simulink library "VIS_LIB"  (Simulink 8.6)
settings: Solver=ode45  StartTime=0.0  StopTime=10.0  RelTol=1e-3
undefined symbols (not defined in the file): AC, SIXOSEM_F_WD_AC_MASTER
libraries: cdsFilt x376, cdsEpicsOut x253, cdsEpicsIn x179, cdsTP x123, VIS_LIB x95, cdsMuxMatrix x91, cdsEpicsStringIn x75, cdsFiltCtrl x72, cdsFunctionCall x70, cdsRms x59, KAGRA_UTIL x25, STATE_BIO_MASTER x5
(part 17 of 38)

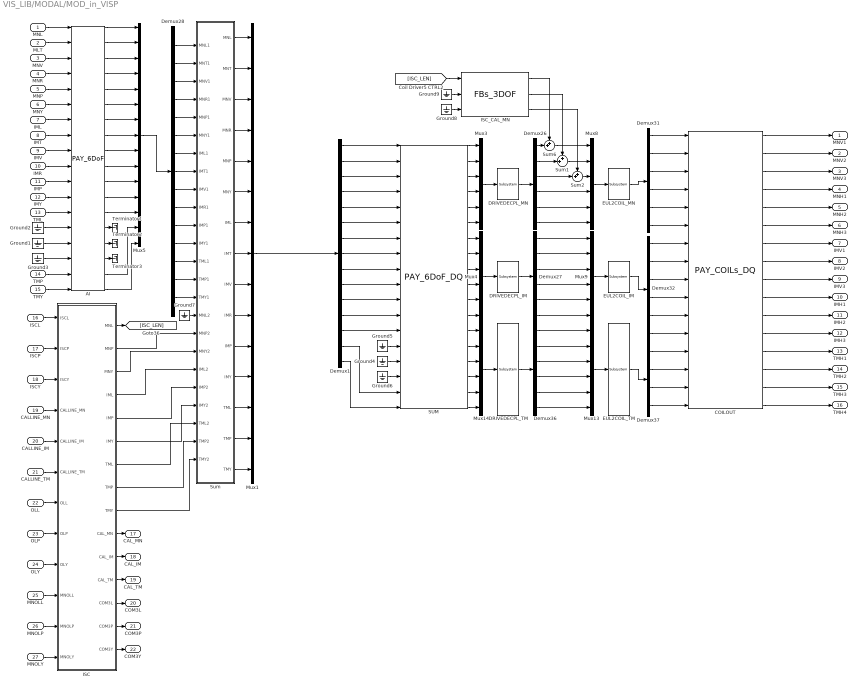
== system VIS_LIB/MODAL/MOD_in_VISP ==
  MNL : Inport
  MLT : Inport  Port=2
  MNV : Inport  Port=3
  MNR : Inport  Port=4
  MNP : Inport  Port=5
  MNY : Inport  Port=6
  IML : Inport  Port=7
  IMT : Inport  Port=8
  IMV : Inport  Port=9
  IMR : Inport  Port=10
  IMP : Inport  Port=11
  IMY : Inport  Port=12
  TML : Inport  Port=13
  TMP : Inport  Port=14
  TMY : Inport  Port=15
  ISCL : Inport  Port=16
  ISCP : Inport  Port=17
  ISCY : Inport  Port=18
  CALLINE_MN : Inport  Port=19
  CALLINE_IM : Inport  Port=20
  CALLINE_TM : Inport  Port=21
  OLL : Inport  Port=22
  OLP : Inport  Port=23
  OLY : Inport  Port=24
  MNOLL : Inport  Port=25
  MNOLP : Inport  Port=26
  MNOLY : Inport  Port=27
  AI : VIS_LIB/UTILs/PAY_6DoF
  COILOUT : VIS_LIB/UTILs/PAY_COILs_DQ
  DRIVEDECPL_IM : cdsMuxMatrix/Subsystem  Tag=cdsMuxMatrix  Description=Any size matrix. Inputs and outputs must be connected using Mux and Demux parts.
      settings: AttributesFormatString=%<Tag>
  DRIVEDECPL_MN : cdsMuxMatrix/Subsystem  Tag=cdsMuxMatrix  Description=Any size matrix. Inputs and outputs must be connected using Mux and Demux parts.
      settings: AttributesFormatString=%<Tag>
  DRIVEDECPL_TM : cdsMuxMatrix/Subsystem  Tag=cdsMuxMatrix  Description=Any size matrix. Inputs and outputs must be connected using Mux and Demux parts.
      settings: AttributesFormatString=%<Tag>
  Demux1 : Demux  Outputs=15
  Demux{26..27,31..32,36} (5 alike) : Demux  Outputs=6
  Demux28 : Demux  Outputs=15
  Demux37 : Demux
  EUL2COIL_IM : cdsMuxMatrix/Subsystem  Tag=cdsMuxMatrix  Description=Any size matrix. Inputs and outputs must be connected using Mux and Demux parts.
      settings: AttributesFormatString=%<Tag>
  EUL2COIL_MN : cdsMuxMatrix/Subsystem  Tag=cdsMuxMatrix  Description=Any size matrix. Inputs and outputs must be connected using Mux and Demux parts.
      settings: AttributesFormatString=%<Tag>
  EUL2COIL_TM : cdsMuxMatrix/Subsystem  Tag=cdsMuxMatrix  Description=Any size matrix. Inputs and outputs must be connected using Mux and Demux parts.
      settings: AttributesFormatString=%<Tag>
  Ground{1..9} (9 alike) : Ground
  ISC : Subsystem
  ISC_CAL_MN : VIS_LIB/UTILs/FBs_3DOF
  Mux1 : Mux  Inputs=15
  Mux{3..4,8..9,13..14} (6 alike) : Mux  Inputs=6
  Mux5 : Mux  Inputs=15
  SUM : VIS_LIB/UTILs/PAY_6DoF_DQ
  Sum : Subsystem
  Sum1 : Sum  Inputs=++|
  Sum2 : Sum  Inputs=++|
  Sum6 : Sum  Inputs=++|
  Terminator1 : Terminator
  Terminator2 : Terminator
  Terminator3 : Terminator
  MNV1 : Outport
  MNV2 : Outport  Port=2
  MNV3 : Outport  Port=3
  MNH1 : Outport  Port=4
  MNH2 : Outport  Port=5
  MNH3 : Outport  Port=6
  IMV1 : Outport  Port=7
  IMV2 : Outport  Port=8
  IMV3 : Outport  Port=9
  IMH1 : Outport  Port=10
  IMH2 : Outport  Port=11
  IMH3 : Outport  Port=12
  TMH1 : Outport  Port=13
  TMH2 : Outport  Port=14
  TMH3 : Outport  Port=15
  TMH4 : Outport  Port=16
  CAL_MN : Outport  Port=17
  CAL_IM : Outport  Port=18
  CAL_TM : Outport  Port=19
  COM3L : Outport  Port=20
  COM3P : Outport  Port=21
  COM3Y : Outport  Port=22
  wires:
  ISC/12(CAL_TM) -> CAL_TM/1
  ISC/11(CAL_IM) -> CAL_IM/1
  ISC/10(CAL_MN) -> CAL_MN/1
  Mux1/1 -> Demux1/1
  Demux1/15 -> SUM/18
  Demux1/14 -> SUM/17
  Demux1/13 -> SUM/13
  Demux1/12 -> SUM/12
  Demux1/10 -> SUM/10
  Demux1/9 -> SUM/9
  Demux1/8 -> SUM/8
  Demux1/7 -> SUM/7
  Demux1/6 -> SUM/6
  Demux1/5 -> SUM/5
  Demux1/4 -> SUM/4
  Demux1/3 -> SUM/3
  Demux1/2 -> SUM/2
  Demux1/1 -> SUM/1
  Ground6/1 -> SUM/16
  Ground4/1 -> SUM/15
  Ground5/1 -> SUM/14
  Demux1/11 -> SUM/11
  Sum/15(TMY) -> Mux1/15
  Sum/14(TMP) -> Mux1/14
  Sum/13(TML) -> Mux1/13
  Sum/12(IMY) -> Mux1/12
  Sum/11(IMP) -> Mux1/11
  Sum/10(IMR) -> Mux1/10
  Sum/9(IMV) -> Mux1/9
  Sum/8(IMT) -> Mux1/8
  Sum/7(IML) -> Mux1/7
  Sum/6(MNY) -> Mux1/6
  Sum/5(MNP) -> Mux1/5
  Sum/4(MNR) -> Mux1/4
  Sum/3(MNV) -> Mux1/3
  Sum/2(MNT) -> Mux1/2
  Sum/1(MNL) -> Mux1/1
  ISCY/1 -> ISC/3(ISCY)
  ISCP/1 -> ISC/2(ISCP)
  CALLINE_MN/1 -> ISC/4(CALLINE_MN)
  CALLINE_IM/1 -> ISC/5(CALLINE_IM)
  CALLINE_TM/1 -> ISC/6(CALLINE_TM)
  ISCL/1 -> ISC/1(ISCL)
  ISC/9(TMY) -> Sum/24(TMY2)
  ISC/8(TMP) -> Sum/23(TMP2)
  ISC/7(TML) -> Sum/22(TML2)
  ISC/6(IMY) -> Sum/21(IMY2)
  ISC/5(IMP) -> Sum/20(IMP2)
  ISC/4(IML) -> Sum/19(IML2)
  Mux5/1 -> Demux28/1
  Demux28/15 -> Sum/15(TMY1)
  Demux28/14 -> Sum/14(TMP1)
  Demux28/13 -> Sum/13(TML1)
  Demux28/12 -> Sum/12(IMY1)
  Demux28/11 -> Sum/11(IMP1)
  Demux28/10 -> Sum/10(IMR1)
  Demux28/9 -> Sum/9(IMV1)
  Demux28/8 -> Sum/8(IMT1)
  Demux28/7 -> Sum/7(IML1)
  Demux28/6 -> Sum/6(MNY1)
  Demux28/5 -> Sum/5(MNP1)
  Demux28/4 -> Sum/4(MNR1)
  Demux28/3 -> Sum/3(MNV1)
  Demux28/2 -> Sum/2(MNT1)
  Demux28/1 -> Sum/1(MNL1)
  AI/18 -> Mux5/15
  AI/17 -> Mux5/14
  AI/13 -> Mux5/13
  AI/12 -> Mux5/12
  AI/11 -> Mux5/11
  AI/10 -> Mux5/10
  AI/9 -> Mux5/9
  AI/8 -> Mux5/8
  AI/7 -> Mux5/7
  AI/6 -> Mux5/6
  AI/5 -> Mux5/5
  AI/4 -> Mux5/4
  AI/3 -> Mux5/3
  AI/2 -> Mux5/2
  AI/1 -> Mux5/1
  AI/16 -> Terminator3/1
  AI/15 -> Terminator2/1
  AI/14 -> Terminator1/1
  SUM/10 -> Mux4/4
  SUM/9 -> Mux4/3
  SUM/8 -> Mux4/2
  SUM/7 -> Mux4/1
  SUM/6 -> Mux3/6
  SUM/5 -> Mux3/5
  SUM/4 -> Mux3/4
  SUM/3 -> Mux3/3
  SUM/2 -> Mux3/2
  SUM/1 -> Mux3/1
  SUM/18 -> Mux14/6
  SUM/17 -> Mux14/5
  SUM/16 -> Mux14/4
  SUM/15 -> Mux14/3
  SUM/14 -> Mux14/2
  SUM/13 -> Mux14/1
  SUM/12 -> Mux4/6
  SUM/11 -> Mux4/5
  COILOUT/16 -> TMH4/1
  COILOUT/15 -> TMH3/1
  COILOUT/14 -> TMH2/1
  COILOUT/13 -> TMH1/1
  COILOUT/12 -> IMH3/1
  COILOUT/11 -> IMH2/1
  COILOUT/10 -> IMH1/1
  COILOUT/9 -> IMV3/1
  COILOUT/8 -> IMV2/1
  COILOUT/7 -> IMV1/1
  COILOUT/6 -> MNH3/1
  COILOUT/5 -> MNH2/1
  COILOUT/4 -> MNH1/1
  COILOUT/3 -> MNV3/1
  COILOUT/2 -> MNV2/1
  COILOUT/1 -> MNV1/1
  Demux37/4 -> COILOUT/16
  Demux37/3 -> COILOUT/15
  Demux37/2 -> COILOUT/14
  Demux37/1 -> COILOUT/13
  Demux32/6 -> COILOUT/12
  Demux32/5 -> COILOUT/11
  Demux32/4 -> COILOUT/10
  Demux32/3 -> COILOUT/9
  Demux32/2 -> COILOUT/8
  Demux32/1 -> COILOUT/7
  Demux31/6 -> COILOUT/6
  Demux31/5 -> COILOUT/5
  Demux31/4 -> COILOUT/4
  Demux31/3 -> COILOUT/3
  Demux31/2 -> COILOUT/2
  Demux31/1 -> COILOUT/1
  Ground3/1 -> AI/16
  Ground1/1 -> AI/15
  Ground2/1 -> AI/14
  TMY/1 -> AI/18
  TMP/1 -> AI/17
  TML/1 -> AI/13
  IMY/1 -> AI/12
  IMP/1 -> AI/11
  IMR/1 -> AI/10
  IMV/1 -> AI/9
  IMT/1 -> AI/8
  IML/1 -> AI/7
  MNY/1 -> AI/6
  MNP/1 -> AI/5
  MNR/1 -> AI/4
  MNV/1 -> AI/3
  MLT/1 -> AI/2
  MNL/1 -> AI/1
  Mux3/1 -> DRIVEDECPL_MN/1
  DRIVEDECPL_MN/1 -> Demux26/1
  Mux4/1 -> DRIVEDECPL_IM/1
  DRIVEDECPL_IM/1 -> Demux27/1
  Mux8/1 -> EUL2COIL_MN/1
  EUL2COIL_MN/1 -> Demux31/1
  Demux26/4 -> Mux8/4
  Demux26/5 -> Mux8/5
  Demux26/6 -> Mux8/6
  Mux9/1 -> EUL2COIL_IM/1
  EUL2COIL_IM/1 -> Demux32/1
  Demux27/1 -> Mux9/1
  Demux27/2 -> Mux9/2
  Demux27/3 -> Mux9/3
  Demux27/4 -> Mux9/4
  Demux27/5 -> Mux9/5
  Demux27/6 -> Mux9/6
  Mux14/1 -> DRIVEDECPL_TM/1
  DRIVEDECPL_TM/1 -> Demux36/1
  Mux13/1 -> EUL2COIL_TM/1
  EUL2COIL_TM/1 -> Demux37/1
  Demux36/1 -> Mux13/1
  Demux36/2 -> Mux13/2
  Demux36/3 -> Mux13/3
  Demux36/4 -> Mux13/4
  Demux36/5 -> Mux13/5
  Demux36/6 -> Mux13/6
  ISC/13(COM3L) -> COM3L/1
  ISC/14(COM3P) -> COM3P/1
  ISC/15(COM3Y) -> COM3Y/1
  OLY/1 -> ISC/9(OLY)
  OLP/1 -> ISC/8(OLP)
  OLL/1 -> ISC/7(OLL)
  MNOLY/1 -> ISC/12(MNOLY)
  MNOLP/1 -> ISC/11(MNOLP)
  MNOLL/1 -> ISC/10(MNOLL)
  Ground7/1 -> Sum/16(MNL2)
  Demux26/1 -> Sum6/2
  Sum6/1 -> Mux8/1
  ISC/1(MNL) -> [ISC_LEN]
  Sum2/1 -> Mux8/3
  Sum1/1 -> Mux8/2
  Demux26/2 -> Sum1/2
  Demux26/3 -> Sum2/2
  [ISC_LEN] -> ISC_CAL_MN/1
  ISC/2(MNP) -> Sum/17(MNP2)
  ISC/3(MNY) -> Sum/18(MNY2)
  ISC_CAL_MN/1 -> Sum6/1
  ISC_CAL_MN/2 -> Sum1/1
  ISC_CAL_MN/3 -> Sum2/1
  Ground8/1 -> ISC_CAL_MN/3
  Ground9/1 -> ISC_CAL_MN/2

== system VIS_LIB/MODAL/MOD_in_VIST ==
  IPL : Inport
  IPT : Inport  Port=2
  IPY : Inport  Port=3
  BFL : Inport  Port=4
  BFT : Inport  Port=5
  BFV : Inport  Port=6
  BFR : Inport  Port=7
  BFP : Inport  Port=8
  BFY : Inport  Port=9
  ISC_MN : Inport  Port=10
  ISC_MN1 : Inport  Port=11
  AI_BF : VIS_LIB/UTILs/FBs_6DOF_DQ
  AI_IP : VIS_LIB/UTILs/FBs_6DOF_DQ
  COILOUT_BF : VIS_LIB/UTILs/6COILs_DQ
  COILOUT_IP : VIS_LIB/UTILs/6COILs_DQ
  DRIVEDECPL_BF : cdsMuxMatrix/Subsystem  Tag=cdsMuxMatrix  Description=Any size matrix. Inputs and outputs must be connected using Mux and Demux parts.
      settings: AttributesFormatString=%<Tag>
  DRIVEDECPL_IP : cdsMuxMatrix/Subsystem  Tag=cdsMuxMatrix  Description=Any size matrix. Inputs and outputs must be connected using Mux and Demux parts.
      settings: AttributesFormatString=%<Tag>
  Demux{29..30,34..35} (4 alike) : Demux  Outputs=6
  EUL2COIL_BF : cdsMuxMatrix/Subsystem  Tag=cdsMuxMatrix  Description=Any size matrix. Inputs and outputs must be connected using Mux and Demux parts.
      settings: AttributesFormatString=%<Tag>
  EUL2COIL_IP : cdsMuxMatrix/Subsystem  Tag=cdsMuxMatrix  Description=Any size matrix. Inputs and outputs must be connected using Mux and Demux parts.
      settings: AttributesFormatString=%<Tag>
  Ground{1,10..11,23} (4 alike) : Ground
  ISC_BF : VIS_LIB/UTILs/FBs_3DOF
  ISC_DRIVEALIGN_BF : VIS_LIB/UTILs/DRIVEALIGN
  ISC_WD : Subsystem
  Mux{6..7,11..12} (4 alike) : Mux  Inputs=6
  SUM_BF : VIS_LIB/UTILs/FBs_6DOF_DQ
  SUM_IP : VIS_LIB/UTILs/FBs_6DOF_DQ
  Sum : Sum  Inputs=|++
  Sum1 : Sum  Inputs=|++
  Sum2 : Sum  Inputs=|++
  Terminator1 : Terminator
  Terminator2 : Terminator
  Terminator3 : Terminator
  IPH1 : Outport
  IPH2 : Outport  Port=2
  IPH3 : Outport  Port=3
  BFV1 : Outport  Port=4
  BFV2 : Outport  Port=5
  BFV3 : Outport  Port=6
  BFH1 : Outport  Port=7
  BFH2 : Outport  Port=8
  BFH3 : Outport  Port=9
  wires:
  AI_BF/4 -> SUM_BF/4
  AI_BF/3 -> SUM_BF/3
  AI_BF/2 -> SUM_BF/2
  Sum/1 -> SUM_BF/1
  AI_IP/6 -> SUM_IP/6
  AI_IP/5 -> SUM_IP/5
  AI_IP/4 -> SUM_IP/4
  AI_IP/3 -> SUM_IP/3
  AI_IP/2 -> SUM_IP/2
  AI_IP/1 -> SUM_IP/1
  SUM_BF/6 -> Mux6/6
  SUM_BF/5 -> Mux6/5
  SUM_BF/4 -> Mux6/4
  SUM_BF/3 -> Mux6/3
  SUM_BF/2 -> Mux6/2
  SUM_BF/1 -> Mux6/1
  SUM_IP/6 -> Mux7/6
  SUM_IP/5 -> Mux7/5
  SUM_IP/4 -> Mux7/4
  SUM_IP/3 -> Mux7/3
  SUM_IP/2 -> Mux7/2
  SUM_IP/1 -> Mux7/1
  AI_BF/1 -> Sum/1
  ISC_MN/1 -> ISC_BF/1
  ISC_DRIVEALIGN_BF/2 -> Sum1/2
  ISC_DRIVEALIGN_BF/3 -> Sum2/2
  ISC_MN1/1 -> ISC_BF/3
  Ground1/1 -> ISC_BF/2
  ISC_DRIVEALIGN_BF/1 -> Sum/2
  BFL/1 -> AI_BF/1
  Demux30/6 -> Mux12/6
  Demux30/5 -> Mux12/5
  Demux30/4 -> Mux12/4
  Demux35/4 -> COILOUT_IP/4
  Demux35/5 -> COILOUT_IP/5
  Demux35/6 -> COILOUT_IP/6
  Ground23/1 -> AI_IP/5
  Ground10/1 -> AI_IP/4
  Ground11/1 -> AI_IP/3
  Demux34/6 -> COILOUT_BF/6
  Demux34/5 -> COILOUT_BF/5
  Demux34/4 -> COILOUT_BF/4
  Demux34/3 -> COILOUT_BF/3
  Demux34/2 -> COILOUT_BF/2
  Demux34/1 -> COILOUT_BF/1
  Demux30/3 -> Mux12/3
  Demux30/2 -> Mux12/2
  Demux30/1 -> Mux12/1
  EUL2COIL_IP/1 -> Demux35/1
  Mux12/1 -> EUL2COIL_IP/1
  Demux29/6 -> Mux11/6
  Demux29/5 -> Mux11/5
  Demux29/4 -> Mux11/4
  Demux29/3 -> Mux11/3
  Demux29/2 -> Mux11/2
  Demux29/1 -> Mux11/1
  EUL2COIL_BF/1 -> Demux34/1
  Mux11/1 -> EUL2COIL_BF/1
  DRIVEDECPL_IP/1 -> Demux30/1
  Mux7/1 -> DRIVEDECPL_IP/1
  DRIVEDECPL_BF/1 -> Demux29/1
  Mux6/1 -> DRIVEDECPL_BF/1
  BFY/1 -> AI_BF/6
  BFP/1 -> AI_BF/5
  BFR/1 -> AI_BF/4
  BFV/1 -> AI_BF/3
  BFT/1 -> AI_BF/2
  IPY/1 -> AI_IP/6
  IPT/1 -> AI_IP/2
  IPL/1 -> AI_IP/1
  COILOUT_BF/4 -> BFH1/1
  COILOUT_BF/2 -> BFV2/1
  COILOUT_BF/6 -> BFH3/1
  COILOUT_BF/5 -> BFH2/1
  COILOUT_BF/3 -> BFV3/1
  COILOUT_BF/1 -> BFV1/1
  COILOUT_IP/6 -> IPH3/1
  COILOUT_IP/4 -> IPH1/1
  COILOUT_IP/5 -> IPH2/1
  Demux35/3 -> COILOUT_IP/3
  Demux35/2 -> COILOUT_IP/2
  Demux35/1 -> COILOUT_IP/1
  COILOUT_IP/1 -> Terminator1/1
  COILOUT_IP/2 -> Terminator2/1
  COILOUT_IP/3 -> Terminator3/1
  Sum1/1 -> SUM_BF/5
  AI_BF/5 -> Sum1/1
  Sum2/1 -> SUM_BF/6
  AI_BF/6 -> Sum2/1
  ISC_BF/1 -> ISC_WD/1(L)
  ISC_BF/2 -> ISC_WD/2(P)
  ISC_BF/3 -> ISC_WD/3(Y)
  ISC_WD/1(LEN) -> ISC_DRIVEALIGN_BF/1
  ISC_WD/2(PIT) -> ISC_DRIVEALIGN_BF/2
  ISC_WD/3(YAW) -> ISC_DRIVEALIGN_BF/3

== system VIS_LIB/MODAL/MOD_in_VIST_with_GAS ==
  IPL : Inport
  IPT : Inport  Port=2
  IPY : Inport  Port=3
  BFL : Inport  Port=4
  BFT : Inport  Port=5
  BFV : Inport  Port=6
  BFR : Inport  Port=7
  BFP : Inport  Port=8
  BFY : Inport  Port=9
  ISC_MN : Inport  Port=10
  F0GASi : Inport  Port=11
  F1GASi : Inport  Port=12
  F2GASi : Inport  Port=13
  F3GASi : Inport  Port=14
  BFGASi : Inport  Port=15
  AI_BF : VIS_LIB/UTILs/FBs_6DOF_DQ
  AI_IP : VIS_LIB/UTILs/FBs_6DOF_DQ
  COILOUT_BF : VIS_LIB/UTILs/7COILs_DQ1
  COILOUT_F{0..3} (4 alike) : VIS_LIB/UTILs/1COIL_DQ
  COILOUT_IP : VIS_LIB/UTILs/6COILs_DQ
  DRIVEDECPL_BF : cdsMuxMatrix/Subsystem  Tag=cdsMuxMatrix  Description=Any size matrix. Inputs and outputs must be connected using Mux and Demux parts.
      settings: AttributesFormatString=%<Tag>
  DRIVEDECPL_IP : cdsMuxMatrix/Subsystem  Tag=cdsMuxMatrix  Description=Any size matrix. Inputs and outputs must be connected using Mux and Demux parts.
      settings: AttributesFormatString=%<Tag>
  Demux{29..30,34..35} (4 alike) : Demux  Outputs=6
  EUL2COIL_BF : cdsMuxMatrix/Subsystem  Tag=cdsMuxMatrix  Description=Any size matrix. Inputs and outputs must be connected using Mux and Demux parts.
      settings: AttributesFormatString=%<Tag>
  EUL2COIL_IP : cdsMuxMatrix/Subsystem  Tag=cdsMuxMatrix  Description=Any size matrix. Inputs and outputs must be connected using Mux and Demux parts.
      settings: AttributesFormatString=%<Tag>
  Ground{1..2,10..11,23} (5 alike) : Ground
  ISC_BF : VIS_LIB/UTILs/FBs_3DOF
  ISC_DRIVEALIGN_BF : VIS_LIB/UTILs/DRIVEALIGN
  Mux{6..7,11..12} (4 alike) : Mux  Inputs=6
  SUM_BF : VIS_LIB/UTILs/FBs_6DOF_DQ
  SUM_IP : VIS_LIB/UTILs/FBs_6DOF_DQ
  Sum : Sum  Inputs=|++
  Terminator{1..5} (5 alike) : Terminator
  IPH1 : Outport
  IPH2 : Outport  Port=2
  IPH3 : Outport  Port=3
  BFV1 : Outport  Port=4
  BFV2 : Outport  Port=5
  BFV3 : Outport  Port=6
  BFH1 : Outport  Port=7
  BFH2 : Outport  Port=8
  BFH3 : Outport  Port=9
  F0GASo : Outport  Port=10
  F1GASo : Outport  Port=11
  F2GASo : Outport  Port=12
  F3GASo : Outport  Port=13
  BFGASo : Outport  Port=14
  wires:
  AI_BF/6 -> SUM_BF/6
  AI_BF/5 -> SUM_BF/5
  AI_BF/4 -> SUM_BF/4
  AI_BF/3 -> SUM_BF/3
  AI_BF/2 -> SUM_BF/2
  Sum/1 -> SUM_BF/1
  AI_IP/6 -> SUM_IP/6
  AI_IP/5 -> SUM_IP/5
  AI_IP/4 -> SUM_IP/4
  AI_IP/3 -> SUM_IP/3
  AI_IP/2 -> SUM_IP/2
  AI_IP/1 -> SUM_IP/1
  SUM_BF/6 -> Mux6/6
  SUM_BF/5 -> Mux6/5
  SUM_BF/4 -> Mux6/4
  SUM_BF/3 -> Mux6/3
  SUM_BF/2 -> Mux6/2
  SUM_BF/1 -> Mux6/1
  SUM_IP/6 -> Mux7/6
  SUM_IP/5 -> Mux7/5
  SUM_IP/4 -> Mux7/4
  SUM_IP/3 -> Mux7/3
  SUM_IP/2 -> Mux7/2
  SUM_IP/1 -> Mux7/1
  AI_BF/1 -> Sum/1
  ISC_MN/1 -> ISC_BF/1
  ISC_DRIVEALIGN_BF/2 -> Terminator4/1
  ISC_DRIVEALIGN_BF/3 -> Terminator5/1
  Ground2/1 -> ISC_BF/3
  Ground1/1 -> ISC_BF/2
  ISC_DRIVEALIGN_BF/1 -> Sum/2
  BFL/1 -> AI_BF/1
  ISC_BF/3 -> ISC_DRIVEALIGN_BF/3
  ISC_BF/2 -> ISC_DRIVEALIGN_BF/2
  ISC_BF/1 -> ISC_DRIVEALIGN_BF/1
  Demux30/6 -> Mux12/6
  Demux30/5 -> Mux12/5
  Demux30/4 -> Mux12/4
  Demux35/4 -> COILOUT_IP/4
  Demux35/5 -> COILOUT_IP/5
  Demux35/6 -> COILOUT_IP/6
  Ground23/1 -> AI_IP/5
  Ground10/1 -> AI_IP/4
  Ground11/1 -> AI_IP/3
  Demux34/6 -> COILOUT_BF/6
  Demux34/5 -> COILOUT_BF/5
  Demux34/4 -> COILOUT_BF/4
  Demux34/3 -> COILOUT_BF/3
  Demux34/2 -> COILOUT_BF/2
  Demux34/1 -> COILOUT_BF/1
  Demux30/3 -> Mux12/3
  Demux30/2 -> Mux12/2
  Demux30/1 -> Mux12/1
  EUL2COIL_IP/1 -> Demux35/1
  Mux12/1 -> EUL2COIL_IP/1
  Demux29/6 -> Mux11/6
  Demux29/5 -> Mux11/5
  Demux29/4 -> Mux11/4
  Demux29/3 -> Mux11/3
  Demux29/2 -> Mux11/2
  Demux29/1 -> Mux11/1
  EUL2COIL_BF/1 -> Demux34/1
  Mux11/1 -> EUL2COIL_BF/1
  DRIVEDECPL_IP/1 -> Demux30/1
  Mux7/1 -> DRIVEDECPL_IP/1
  DRIVEDECPL_BF/1 -> Demux29/1
  Mux6/1 -> DRIVEDECPL_BF/1
  BFY/1 -> AI_BF/6
  BFP/1 -> AI_BF/5
  BFR/1 -> AI_BF/4
  BFV/1 -> AI_BF/3
  BFT/1 -> AI_BF/2
  IPY/1 -> AI_IP/6
  IPT/1 -> AI_IP/2
  IPL/1 -> AI_IP/1
  COILOUT_BF/4 -> BFH1/1
  COILOUT_BF/2 -> BFV2/1
  COILOUT_BF/6 -> BFH3/1
  COILOUT_BF/5 -> BFH2/1
  COILOUT_BF/3 -> BFV3/1
  COILOUT_BF/1 -> BFV1/1
  COILOUT_IP/6 -> IPH3/1
  COILOUT_IP/4 -> IPH1/1
  COILOUT_IP/5 -> IPH2/1
  Demux35/3 -> COILOUT_IP/3
  Demux35/2 -> COILOUT_IP/2
  Demux35/1 -> COILOUT_IP/1
  COILOUT_IP/1 -> Terminator1/1
  COILOUT_IP/2 -> Terminator2/1
  COILOUT_IP/3 -> Terminator3/1
  F0GASi/1 -> COILOUT_F0/1
  COILOUT_F0/1 -> F0GASo/1
  F1GASi/1 -> COILOUT_F1/1
  COILOUT_F1/1 -> F1GASo/1
  COILOUT_F2/1 -> F2GASo/1
  F2GASi/1 -> COILOUT_F2/1
  F3GASi/1 -> COILOUT_F3/1
  COILOUT_F3/1 -> F3GASo/1
  BFGASi/1 -> COILOUT_BF/7
  COILOUT_BF/7 -> BFGASo/1

== system VIS_LIB/MODAL/SENSDIAG ==
  BF : Subsystem
  GAS : Subsystem
  IM : Subsystem
  IP : Subsystem
  MN : Subsystem
  TM : Subsystem

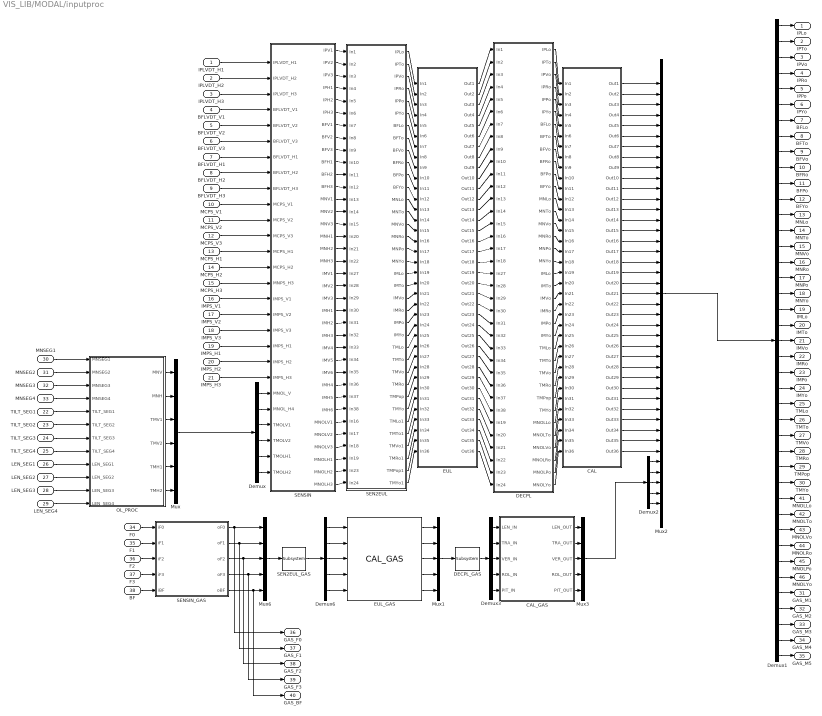
== system VIS_LIB/MODAL/inputproc ==
  IPLVDT_H1 : Inport
  IPLVDT_H2 : Inport  Port=2
  IPLVDT_H3 : Inport  Port=3
  BFLVDT_V1 : Inport  Port=4
  BFLVDT_V2 : Inport  Port=5
  BFLVDT_V3 : Inport  Port=6
  BFLVDT_H1 : Inport  Port=7
  BFLVDT_H2 : Inport  Port=8
  BFLVDT_H3 : Inport  Port=9
  MCPS_V1 : Inport  Port=10
  MCPS_V2 : Inport  Port=11
  MCPS_V3 : Inport  Port=12
  MCPS_H1 : Inport  Port=13
  MCPS_H2 : Inport  Port=14
  MCPS_H3 : Inport  Port=15
  IMPS_V1 : Inport  Port=16
  IMPS_V2 : Inport  Port=17
  IMPS_V3 : Inport  Port=18
  IMPS_H1 : Inport  Port=19
  IMPS_H2 : Inport  Port=20
  IMPS_H3 : Inport  Port=21
  TILT_SEG1 : Inport  Port=22
  TILT_SEG2 : Inport  Port=23
  TILT_SEG3 : Inport  Port=24
  TILT_SEG4 : Inport  Port=25
  LEN_SEG1 : Inport  Port=26
  LEN_SEG2 : Inport  Port=27
  LEN_SEG3 : Inport  Port=28
  LEN_SEG4 : Inport  Port=29
  MNSEG1 : Inport  Port=30
  MNSEG2 : Inport  Port=31
  MNSEG3 : Inport  Port=32
  MNSEG4 : Inport  Port=33
  F0 : Inport  Port=34
  F1 : Inport  Port=35
  F2 : Inport  Port=36
  F3 : Inport  Port=37
  BF : Inport  Port=38
  CAL : Subsystem
  CAL_GAS : Subsystem
  DECPL : Subsystem
  DECPL_GAS : cdsMuxMatrix/Subsystem  Tag=cdsMuxMatrix  Description=Any size matrix. Inputs and outputs must be connected using Mux and Demux parts.
      settings: AttributesFormatString=%<Tag>
  Demux : Demux  Outputs=6
  Demux1 : Demux  Outputs=41
  Demux2 : Demux  Outputs=5
  Demux3 : Demux  Outputs=5
  Demux6 : Demux  Outputs=5
  EUL : Subsystem
  EUL_GAS : VIS_LIB/MODAL/inputproc/CAL_GAS
  Mux : Mux  Inputs=6
  Mux1 : Mux  Inputs=5
  Mux2 : Mux  Inputs=41
  Mux3 : Mux  Inputs=5
  Mux6 : Mux  Inputs=5
  OL_PROC : Subsystem
  SEN2EUL : Subsystem
  SEN2EUL_GAS : cdsMuxMatrix/Subsystem  Tag=cdsMuxMatrix  Description=Any size matrix. Inputs and outputs must be connected using Mux and Demux parts.
      settings: AttributesFormatString=%<Tag>
  SENSIN : Subsystem
  SENSIN_GAS : Subsystem
  IPLo : Outport
  IPTo : Outport  Port=2
  IPVo : Outport  Port=3
  IPRo : Outport  Port=4
  IPPo : Outport  Port=5
  IPYo : Outport  Port=6
  BFLo : Outport  Port=7
  BFTo : Outport  Port=8
  BFVo : Outport  Port=9
  BFRo : Outport  Port=10
  BFPo : Outport  Port=11
  BFYo : Outport  Port=12
  MNLo : Outport  Port=13
  MNTo : Outport  Port=14
  MNVo : Outport  Port=15
  MNRo : Outport  Port=16
  MNPo : Outport  Port=17
  MNYo : Outport  Port=18
  IMLo : Outport  Port=19
  IMTo : Outport  Port=20
  IMVo : Outport  Port=21
  IMRo : Outport  Port=22
  IMPo : Outport  Port=23
  IMYo : Outport  Port=24
  TMLo : Outport  Port=25
  TMTo : Outport  Port=26
  TMVo : Outport  Port=27
  TMRo : Outport  Port=28
  TMPop : Outport  Port=29
  TMYo : Outport  Port=30
  GAS_M1 : Outport  Port=31
  GAS_M2 : Outport  Port=32
  GAS_M3 : Outport  Port=33
  GAS_M4 : Outport  Port=34
  GAS_M5 : Outport  Port=35
  GAS_F0 : Outport  Port=36
  GAS_F1 : Outport  Port=37
  GAS_F2 : Outport  Port=38
  GAS_F3 : Outport  Port=39
  GAS_BF : Outport  Port=40
  MNOLLo : Outport  Port=41
  MNOLTo : Outport  Port=42
  MNOLVo : Outport  Port=43
  MNOLRo : Outport  Port=44
  MNOLPo : Outport  Port=45
  MNOLYo : Outport  Port=46
  wires:
  IPLVDT_H1/1 -> SENSIN/1(IPLVDT_H1)
  IPLVDT_H2/1 -> SENSIN/2(IPLVDT_H2)
  IPLVDT_H3/1 -> SENSIN/3(IPLVDT_H3)
  BFLVDT_V1/1 -> SENSIN/4(BFLVDT_V1)
  BFLVDT_V2/1 -> SENSIN/5(BFLVDT_V2)
  BFLVDT_V3/1 -> SENSIN/6(BFLVDT_V3)
  BFLVDT_H1/1 -> SENSIN/7(BFLVDT_H1)
  BFLVDT_H2/1 -> SENSIN/8(BFLVDT_H2)
  BFLVDT_H3/1 -> SENSIN/9(BFLVDT_H3)
  MCPS_V1/1 -> SENSIN/10(MCPS_V1)
  MCPS_V2/1 -> SENSIN/11(MCPS_V2)
  MCPS_V3/1 -> SENSIN/12(MCPS_V3)
  MCPS_H1/1 -> SENSIN/13(MCPS_H1)
  MCPS_H2/1 -> SENSIN/14(MCPS_H2)
  MCPS_H3/1 -> SENSIN/15(MNPS_H3)
  IMPS_V1/1 -> SENSIN/16(IMPS_V1)
  IMPS_V2/1 -> SENSIN/17(IMPS_V2)
  IMPS_V3/1 -> SENSIN/18(IMPS_V3)
  IMPS_H1/1 -> SENSIN/19(IMPS_H1)
  IMPS_H2/1 -> SENSIN/20(IMPS_H2)
  IMPS_H3/1 -> SENSIN/21(IMPS_H3)
  TILT_SEG1/1 -> OL_PROC/5(TILT_SEG1)
  TILT_SEG2/1 -> OL_PROC/6(TILT_SEG2)
  TILT_SEG3/1 -> OL_PROC/7(TILT_SEG3)
  TILT_SEG4/1 -> OL_PROC/8(TILT_SEG4)
  LEN_SEG1/1 -> OL_PROC/9(LEN_SEG1)
  LEN_SEG2/1 -> OL_PROC/10(LEN_SEG2)
  LEN_SEG3/1 -> OL_PROC/11(LEN_SEG3)
  LEN_SEG4/1 -> OL_PROC/12(LEN_SEG4)
  OL_PROC/1(MNV) -> Mux/1
  OL_PROC/2(MNH) -> Mux/2
  OL_PROC/3(TMV1) -> Mux/3
  OL_PROC/4(TMV2) -> Mux/4
  OL_PROC/5(TMH1) -> Mux/5
  OL_PROC/6(TMH2) -> Mux/6
  Demux/1 -> SENSIN/22(MNOL_V)
  Demux/2 -> SENSIN/23(MNOL_H4)
  Demux/3 -> SENSIN/24(TMOLV1)
  Demux/4 -> SENSIN/25(TMOLV2)
  Demux/5 -> SENSIN/26(TMOLH1)
  Demux/6 -> SENSIN/27(TMOLH2)
  Mux/1 -> Demux/1
  MNSEG1/1 -> OL_PROC/1(MNSEG1)
  MNSEG2/1 -> OL_PROC/2(MNSEG2)
  MNSEG3/1 -> OL_PROC/3(MNSEG3)
  MNSEG4/1 -> OL_PROC/4(MNSEG4)
  Mux2/1 -> Demux1/1
  Demux1/1 -> IPLo/1
  Demux1/2 -> IPTo/1
  Demux1/3 -> IPVo/1
  Demux1/4 -> IPRo/1
  Demux1/5 -> IPPo/1
  Demux1/6 -> IPYo/1
  Demux1/7 -> BFLo/1
  Demux1/8 -> BFTo/1
  Demux1/9 -> BFVo/1
  Demux1/10 -> BFRo/1
  Demux1/11 -> BFPo/1
  Demux1/12 -> BFYo/1
  Demux1/13 -> MNLo/1
  Demux1/14 -> MNTo/1
  Demux1/15 -> MNVo/1
  Demux1/16 -> MNRo/1
  Demux1/17 -> MNPo/1
  Demux1/18 -> MNYo/1
  Demux1/19 -> IMLo/1
  Demux1/20 -> IMTo/1
  Demux1/21 -> IMVo/1
  Demux1/22 -> IMRo/1
  Demux1/23 -> IMPo/1
  Demux1/24 -> IMYo/1
  Demux1/25 -> TMLo/1
  Demux1/26 -> TMTo/1
  Demux1/27 -> TMVo/1
  Demux1/28 -> TMRo/1
  Demux1/29 -> TMPop/1
  Demux1/30 -> TMYo/1
  F0/1 -> SENSIN_GAS/1(iF0)
  F1/1 -> SENSIN_GAS/2(iF1)
  F2/1 -> SENSIN_GAS/3(iF2)
  F3/1 -> SENSIN_GAS/4(iF3)
  BF/1 -> SENSIN_GAS/5(iBF)
  SEN2EUL_GAS/1 -> Demux6/1
  Mux6/1 -> SEN2EUL_GAS/1
  SENSIN_GAS/1(oF0) -> GAS_F0/1, Mux6/1
  SENSIN_GAS/2(oF1) -> GAS_F1/1, Mux6/2
  SENSIN_GAS/3(oF2) -> GAS_F2/1, Mux6/3
  SENSIN_GAS/4(oF3) -> GAS_F3/1, Mux6/4
  SENSIN_GAS/5(oBF) -> GAS_BF/1, Mux6/5
  DECPL_GAS/1 -> Demux3/1
  Mux1/1 -> DECPL_GAS/1
  Demux3/1 -> CAL_GAS/1(LEN_IN)
  Demux3/2 -> CAL_GAS/2(TRA_IN)
  Demux3/3 -> CAL_GAS/3(VER_IN)
  Demux3/4 -> CAL_GAS/4(ROL_IN)
  Demux3/5 -> CAL_GAS/5(PIT_IN)
  DECPL/1(IPLo) -> CAL/1(In1)
  DECPL/2(IPTo) -> CAL/2(In2)
  DECPL/3(IPVo) -> CAL/3(In3)
  DECPL/4(IPRo) -> CAL/4(In4)
  DECPL/5(IPPo) -> CAL/5(In5)
  DECPL/6(IPYo) -> CAL/6(In6)
  DECPL/7(BFLo) -> CAL/7(In7)
  DECPL/8(BFTo) -> CAL/8(In8)
  DECPL/9(BFVo) -> CAL/9(In9)
  DECPL/10(BFRo) -> CAL/10(In10)
  DECPL/11(BFPo) -> CAL/11(In11)
  DECPL/12(BFYo) -> CAL/12(In12)
  DECPL/13(MNLo) -> CAL/13(In13)
  DECPL/14(MNTo) -> CAL/14(In14)
  DECPL/15(MNVo) -> CAL/15(In15)
  DECPL/16(MNRo) -> CAL/16(In16)
  DECPL/17(MNPo) -> CAL/17(In17)
  DECPL/18(MNYo) -> CAL/18(In18)
  DECPL/19(IMLo) -> CAL/19(In19)
  DECPL/20(IMTo) -> CAL/20(In20)
  DECPL/21(IMVo) -> CAL/21(In21)
  DECPL/22(IMRo) -> CAL/22(In22)
  DECPL/23(IMPo) -> CAL/23(In23)
  DECPL/24(IMYo) -> CAL/24(In24)
  DECPL/25(TMLo) -> CAL/25(In25)
  DECPL/26(TMTo) -> CAL/26(In26)
  DECPL/27(TMVo) -> CAL/27(In27)
  DECPL/28(TMRo) -> CAL/28(In28)
  DECPL/29(TMPop) -> CAL/29(In29)
  DECPL/30(TMYo) -> CAL/30(In30)
  CAL_GAS/1(LEN_OUT) -> Mux3/1
  CAL_GAS/2(TRA_OUT) -> Mux3/2
  CAL_GAS/3(VER_OUT) -> Mux3/3
  CAL_GAS/4(ROL_OUT) -> Mux3/4
  CAL_GAS/5(PIT_OUT) -> Mux3/5
  Mux3/1 -> Demux2/1
  SEN2EUL/1(IPLo) -> EUL/1(In1)
  SEN2EUL/2(IPTo) -> EUL/2(In2)
  SEN2EUL/3(IPVo) -> EUL/3(In3)
  SEN2EUL/4(IPRo) -> EUL/4(In4)
  SEN2EUL/5(IPPo) -> EUL/5(In5)
  SEN2EUL/6(IPYo) -> EUL/6(In6)
  SEN2EUL/7(BFLo) -> EUL/7(In7)
  SEN2EUL/8(BFTo) -> EUL/8(In8)
  SEN2EUL/9(BFVo) -> EUL/9(In9)
  SEN2EUL/10(BFRo) -> EUL/10(In10)
  SEN2EUL/11(BFPo) -> EUL/11(In11)
  SEN2EUL/12(BFYo) -> EUL/12(In12)
  SEN2EUL/13(MNLo) -> EUL/13(In13)
  SEN2EUL/14(MNTo) -> EUL/14(In14)
  SEN2EUL/15(MNVo) -> EUL/15(In15)
  SEN2EUL/16(MNRo) -> EUL/16(In16)
  SEN2EUL/17(MNPo) -> EUL/17(In17)
  SEN2EUL/18(MNYo) -> EUL/18(In18)
  SEN2EUL/19(IMLo) -> EUL/19(In19)
  SEN2EUL/20(IMTo) -> EUL/20(In20)
  SEN2EUL/21(IMVo) -> EUL/21(In21)
  SEN2EUL/22(IMRo) -> EUL/22(In22)
  SEN2EUL/23(IMPo) -> EUL/23(In23)
  SEN2EUL/24(IMYo) -> EUL/24(In24)
  SEN2EUL/25(TMLo) -> EUL/25(In25)
  SEN2EUL/26(TMTo) -> EUL/26(In26)
  SEN2EUL/27(TMVo) -> EUL/27(In27)
  SEN2EUL/28(TMRo) -> EUL/28(In28)
  SEN2EUL/29(TMPop) -> EUL/29(In29)
  SEN2EUL/30(TMYo) -> EUL/30(In30)
  EUL/1(Out1) -> DECPL/1(In1)
  EUL/2(Out2) -> DECPL/2(In2)
  EUL/3(Out3) -> DECPL/3(In3)
  EUL/4(Out4) -> DECPL/4(In4)
  EUL/5(Out5) -> DECPL/5(In5)
  EUL/6(Out6) -> DECPL/6(In6)
  EUL/7(Out7) -> DECPL/7(In7)
  EUL/8(Out8) -> DECPL/8(In8)
  EUL/9(Out9) -> DECPL/9(In9)
  EUL/10(Out10) -> DECPL/10(In10)
  EUL/11(Out11) -> DECPL/11(In11)
  EUL/12(Out12) -> DECPL/12(In12)
  EUL/13(Out13) -> DECPL/13(In13)
  EUL/14(Out14) -> DECPL/14(In14)
  EUL/15(Out15) -> DECPL/15(In15)
  EUL/16(Out16) -> DECPL/16(In16)
  EUL/17(Out17) -> DECPL/17(In17)
  EUL/18(Out18) -> DECPL/18(In18)
  EUL/19(Out19) -> DECPL/19(In27)
  EUL/20(Out20) -> DECPL/20(In28)
  EUL/21(Out21) -> DECPL/21(In29)
  EUL/22(Out22) -> DECPL/22(In30)
  EUL/23(Out23) -> DECPL/23(In31)
  EUL/24(Out24) -> DECPL/24(In32)
  EUL/25(Out25) -> DECPL/25(In33)
  EUL/26(Out26) -> DECPL/26(In34)
  EUL/27(Out27) -> DECPL/27(In35)
  EUL/28(Out28) -> DECPL/28(In36)
  EUL/29(Out29) -> DECPL/29(In37)
  EUL/30(Out30) -> DECPL/30(In38)
  Demux6/1 -> EUL_GAS/1
  Demux6/2 -> EUL_GAS/2
  Demux6/3 -> EUL_GAS/3
  Demux6/4 -> EUL_GAS/4
  Demux6/5 -> EUL_GAS/5
  EUL_GAS/1 -> Mux1/1
  EUL_GAS/2 -> Mux1/2
  EUL_GAS/3 -> Mux1/3
  EUL_GAS/4 -> Mux1/4
  EUL_GAS/5 -> Mux1/5
  SENSIN/1(IPV1) -> SEN2EUL/1(In1)
  SENSIN/2(IPV2) -> SEN2EUL/2(In2)
  SENSIN/3(IPV3) -> SEN2EUL/3(In3)
  SENSIN/4(IPH1) -> SEN2EUL/4(In4)
  SENSIN/5(IPH2) -> SEN2EUL/5(In5)
  SENSIN/6(IPH3) -> SEN2EUL/6(In6)
  SENSIN/7(BFV1) -> SEN2EUL/7(In7)
  SENSIN/8(BFV2) -> SEN2EUL/8(In8)
  SENSIN/9(BFV3) -> SEN2EUL/9(In9)
  SENSIN/10(BFH1) -> SEN2EUL/10(In10)
  SENSIN/11(BFH2) -> SEN2EUL/11(In11)
  SENSIN/12(BFH3) -> SEN2EUL/12(In12)
  SENSIN/13(MNV1) -> SEN2EUL/13(In13)
  SENSIN/14(MNV2) -> SEN2EUL/14(In14)
  SENSIN/15(MNV3) -> SEN2EUL/15(In15)
  SENSIN/16(MNH1) -> SEN2EUL/16(In20)
  SENSIN/17(MNH2) -> SEN2EUL/17(In21)
  SENSIN/18(MNH3) -> SEN2EUL/18(In22)
  SENSIN/19(IMV1) -> SEN2EUL/19(In27)
  SENSIN/20(IMV2) -> SEN2EUL/20(In28)
  SENSIN/21(IMV3) -> SEN2EUL/21(In29)
  SENSIN/22(IMH1) -> SEN2EUL/22(In30)
  SENSIN/23(IMH2) -> SEN2EUL/23(In31)
  SENSIN/24(IMH3) -> SEN2EUL/24(In32)
  SENSIN/25(IMV4) -> SEN2EUL/25(In33)
  SENSIN/26(IMV5) -> SEN2EUL/26(In34)
  SENSIN/27(IMV6) -> SEN2EUL/27(In35)
  SENSIN/28(IMH4) -> SEN2EUL/28(In36)
  SENSIN/29(IMH5) -> SEN2EUL/29(In37)
  SENSIN/30(IMH6) -> SEN2EUL/30(In38)
  SENSIN/31(MNOLV1) -> SEN2EUL/31(In16)
  SENSIN/32(MNOLV2) -> SEN2EUL/32(In17)
  SENSIN/33(MNOLV3) -> SEN2EUL/33(In18)
  SENSIN/34(MNOLH1) -> SEN2EUL/34(In19)
  SENSIN/35(MNOLH2) -> SEN2EUL/35(In23)
  SENSIN/36(MNOLH3) -> SEN2EUL/36(In24)
  SEN2EUL/31(TMLo1) -> EUL/31(In31)
  SEN2EUL/32(TMTo1) -> EUL/32(In32)
  SEN2EUL/33(TMVo1) -> EUL/33(In33)
  SEN2EUL/34(TMRo1) -> EUL/34(In34)
  SEN2EUL/35(TMPop1) -> EUL/35(In35)
  SEN2EUL/36(TMYo1) -> EUL/36(In36)
  EUL/31(Out31) -> DECPL/31(In19)
  EUL/32(Out32) -> DECPL/32(In20)
  EUL/33(Out33) -> DECPL/33(In21)
  EUL/34(Out34) -> DECPL/34(In22)
  EUL/35(Out35) -> DECPL/35(In23)
  EUL/36(Out36) -> DECPL/36(In24)
  DECPL/31(MNOLLo) -> CAL/31(In31)
  DECPL/32(MNOLTo) -> CAL/32(In32)
  DECPL/33(MNOLVo) -> CAL/33(In33)
  DECPL/34(MNOLRo) -> CAL/34(In34)
  DECPL/35(MNOLPo) -> CAL/35(In35)
  DECPL/36(MNOLYo) -> CAL/36(In36)
  CAL/1(Out1) -> Mux2/1
  CAL/2(Out2) -> Mux2/2
  CAL/3(Out3) -> Mux2/3
  CAL/4(Out4) -> Mux2/4
  CAL/5(Out5) -> Mux2/5
  CAL/6(Out6) -> Mux2/6
  CAL/7(Out7) -> Mux2/7
  CAL/8(Out8) -> Mux2/8
  CAL/9(Out9) -> Mux2/9
  CAL/10(Out10) -> Mux2/10
  CAL/11(Out11) -> Mux2/11
  CAL/12(Out12) -> Mux2/12
  CAL/13(Out13) -> Mux2/13
  CAL/14(Out14) -> Mux2/14
  CAL/15(Out15) -> Mux2/15
  CAL/16(Out16) -> Mux2/16
  CAL/17(Out17) -> Mux2/17
  CAL/18(Out18) -> Mux2/18
  CAL/19(Out19) -> Mux2/19
  CAL/20(Out20) -> Mux2/20
  CAL/21(Out21) -> Mux2/21
  CAL/22(Out22) -> Mux2/22
  CAL/23(Out23) -> Mux2/23
  CAL/24(Out24) -> Mux2/24
  CAL/25(Out25) -> Mux2/25
  CAL/26(Out26) -> Mux2/26
  CAL/27(Out27) -> Mux2/27
  CAL/28(Out28) -> Mux2/28
  CAL/29(Out29) -> Mux2/29
  CAL/30(Out30) -> Mux2/30
  CAL/31(Out31) -> Mux2/31
  CAL/32(Out32) -> Mux2/32
  CAL/33(Out33) -> Mux2/33
  CAL/34(Out34) -> Mux2/34
  CAL/35(Out35) -> Mux2/35
  CAL/36(Out36) -> Mux2/36
  Demux2/1 -> Mux2/37
  Demux2/2 -> Mux2/38
  Demux2/3 -> Mux2/39
  Demux2/4 -> Mux2/40
  Demux2/5 -> Mux2/41
  Demux1/37 -> GAS_M1/1
  Demux1/38 -> GAS_M2/1
  Demux1/39 -> GAS_M3/1
  Demux1/40 -> GAS_M4/1
  Demux1/41 -> GAS_M5/1
  Demux1/31 -> MNOLLo/1
  Demux1/32 -> MNOLTo/1
  Demux1/33 -> MNOLVo/1
  Demux1/34 -> MNOLRo/1
  Demux1/35 -> MNOLPo/1
  Demux1/36 -> MNOLYo/1

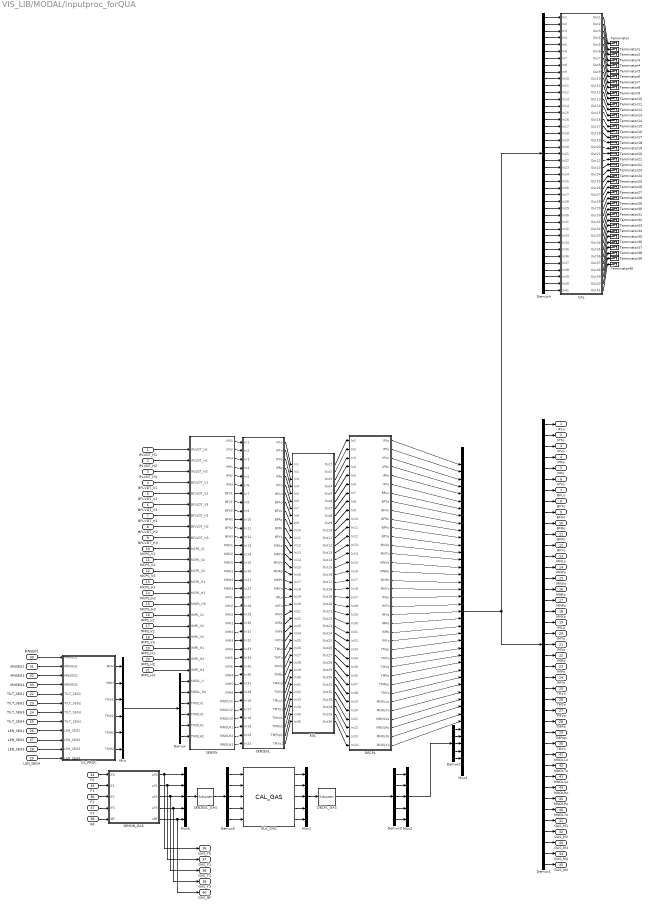
== system VIS_LIB/MODAL/inputproc_forQUA ==
  IPLVDT_H1 : Inport
  IPLVDT_H2 : Inport  Port=2
  IPLVDT_H3 : Inport  Port=3
  BFLVDT_V1 : Inport  Port=4
  BFLVDT_V2 : Inport  Port=5
  BFLVDT_V3 : Inport  Port=6
  BFLVDT_H1 : Inport  Port=7
  BFLVDT_H2 : Inport  Port=8
  BFLVDT_H3 : Inport  Port=9
  MCPS_V1 : Inport  Port=10
  MCPS_V2 : Inport  Port=11
  MCPS_V3 : Inport  Port=12
  MCPS_H1 : Inport  Port=13
  MCPS_H2 : Inport  Port=14
  MCPS_H3 : Inport  Port=15
  IMPS_V1 : Inport  Port=16
  IMPS_V2 : Inport  Port=17
  IMPS_V3 : Inport  Port=18
  IMPS_H1 : Inport  Port=19
  IMPS_H2 : Inport  Port=20
  IMPS_H3 : Inport  Port=21
  TILT_SEG1 : Inport  Port=22
  TILT_SEG2 : Inport  Port=23
  TILT_SEG3 : Inport  Port=24
  TILT_SEG4 : Inport  Port=25
  LEN_SEG1 : Inport  Port=26
  LEN_SEG2 : Inport  Port=27
  LEN_SEG3 : Inport  Port=28
  LEN_SEG4 : Inport  Port=29
  MNSEG1 : Inport  Port=30
  MNSEG2 : Inport  Port=31
  MNSEG3 : Inport  Port=32
  MNSEG4 : Inport  Port=33
  F0 : Inport  Port=34
  F1 : Inport  Port=35
  F2 : Inport  Port=36
  F3 : Inport  Port=37
  BF : Inport  Port=38
  CAL : Subsystem
  DECPL : Subsystem
  DECPL_GAS : cdsMuxMatrix/Subsystem  Tag=cdsMuxMatrix  Description=Any size matrix. Inputs and outputs must be connected using Mux and Demux parts.
      settings: AttributesFormatString=%<Tag>
  Demux : Demux  Outputs=6
  Demux1 : Demux  Outputs=41
  Demux2 : Demux  Outputs=5
  Demux3 : Demux  Outputs=5
  Demux4 : Demux  Outputs=41
  Demux6 : Demux  Outputs=5
  EUL : Subsystem
  EUL_GAS : VIS_LIB/MODAL/inputproc/CAL_GAS
  Mux : Mux  Inputs=6
  Mux1 : Mux  Inputs=5
  Mux2 : Mux  Inputs=41
  Mux3 : Mux  Inputs=5
  Mux6 : Mux  Inputs=5
  OL_PROC : Subsystem
  SEN2EUL : Subsystem
  SEN2EUL_GAS : cdsMuxMatrix/Subsystem  Tag=cdsMuxMatrix  Description=Any size matrix. Inputs and outputs must be connected using Mux and Demux parts.
      settings: AttributesFormatString=%<Tag>
  SENSIN : Subsystem
  SENSIN_GAS : Subsystem
  Terminator{,1..40} (41 alike) : Terminator
  IPLo : Outport
  IPTo : Outport  Port=2
  IPVo : Outport  Port=3
  IPRo : Outport  Port=4
  IPPo : Outport  Port=5
  IPYo : Outport  Port=6
  BFLo : Outport  Port=7
  BFTo : Outport  Port=8
  BFVo : Outport  Port=9
  BFRo : Outport  Port=10
  BFPo : Outport  Port=11
  BFYo : Outport  Port=12
  MNLo : Outport  Port=13
  MNTo : Outport  Port=14
  MNVo : Outport  Port=15
  MNRo : Outport  Port=16
  MNPo : Outport  Port=17
  MNYo : Outport  Port=18
  IMLo : Outport  Port=19
  IMTo : Outport  Port=20
  IMVo : Outport  Port=21
  IMRo : Outport  Port=22
  IMPo : Outport  Port=23
  IMYo : Outport  Port=24
  TMLo : Outport  Port=25
  TMTo : Outport  Port=26
  TMVo : Outport  Port=27
  TMRo : Outport  Port=28
  TMPop : Outport  Port=29
  TMYo : Outport  Port=30
  GAS_M1 : Outport  Port=31
  GAS_M2 : Outport  Port=32
  GAS_M3 : Outport  Port=33
  GAS_M4 : Outport  Port=34
  GAS_M5 : Outport  Port=35
  GAS_F0 : Outport  Port=36
  GAS_F1 : Outport  Port=37
  GAS_F2 : Outport  Port=38
  GAS_F3 : Outport  Port=39
  GAS_BF : Outport  Port=40
  MNOLLo : Outport  Port=41
  MNOLTo : Outport  Port=42
  MNOLVo : Outport  Port=43
  MNOLRo : Outport  Port=44
  MNOLPo : Outport  Port=45
  MNOLYo : Outport  Port=46
  wires:
  IPLVDT_H1/1 -> SENSIN/1(IPLVDT_H1)
  IPLVDT_H2/1 -> SENSIN/2(IPLVDT_H2)
  IPLVDT_H3/1 -> SENSIN/3(IPLVDT_H3)
  BFLVDT_V1/1 -> SENSIN/4(BFLVDT_V1)
  BFLVDT_V2/1 -> SENSIN/5(BFLVDT_V2)
  BFLVDT_V3/1 -> SENSIN/6(BFLVDT_V3)
  BFLVDT_H1/1 -> SENSIN/7(BFLVDT_H1)
  BFLVDT_H2/1 -> SENSIN/8(BFLVDT_H2)
  BFLVDT_H3/1 -> SENSIN/9(BFLVDT_H3)
  MCPS_V1/1 -> SENSIN/10(MCPS_V1)
  MCPS_V2/1 -> SENSIN/11(MCPS_V2)
  MCPS_V3/1 -> SENSIN/12(MCPS_V3)
  MCPS_H1/1 -> SENSIN/13(MCPS_H1)
  MCPS_H2/1 -> SENSIN/14(MCPS_H2)
  MCPS_H3/1 -> SENSIN/15(MNPS_H3)
  IMPS_V1/1 -> SENSIN/16(IMPS_V1)
  IMPS_V2/1 -> SENSIN/17(IMPS_V2)
  IMPS_V3/1 -> SENSIN/18(IMPS_V3)
  IMPS_H1/1 -> SENSIN/19(IMPS_H1)
  IMPS_H2/1 -> SENSIN/20(IMPS_H2)
  IMPS_H3/1 -> SENSIN/21(IMPS_H3)
  TILT_SEG1/1 -> OL_PROC/5(TILT_SEG1)
  TILT_SEG2/1 -> OL_PROC/6(TILT_SEG2)
  TILT_SEG3/1 -> OL_PROC/7(TILT_SEG3)
  TILT_SEG4/1 -> OL_PROC/8(TILT_SEG4)
  LEN_SEG1/1 -> OL_PROC/9(LEN_SEG1)
  LEN_SEG2/1 -> OL_PROC/10(LEN_SEG2)
  LEN_SEG3/1 -> OL_PROC/11(LEN_SEG3)
  LEN_SEG4/1 -> OL_PROC/12(LEN_SEG4)
  OL_PROC/1(MNV) -> Mux/1
  OL_PROC/2(MNH) -> Mux/2
  OL_PROC/3(TMV1) -> Mux/3
  OL_PROC/4(TMV2) -> Mux/4
  OL_PROC/5(TMH1) -> Mux/5
  OL_PROC/6(TMH2) -> Mux/6
  Demux/1 -> SENSIN/22(MNOL_V)
  Demux/2 -> SENSIN/23(MNOL_H4)
  Demux/3 -> SENSIN/24(TMOLV1)
  Demux/4 -> SENSIN/25(TMOLV2)
  Demux/5 -> SENSIN/26(TMOLH1)
  Demux/6 -> SENSIN/27(TMOLH2)
  Mux/1 -> Demux/1
  MNSEG1/1 -> OL_PROC/1(MNSEG1)
  MNSEG2/1 -> OL_PROC/2(MNSEG2)
  MNSEG3/1 -> OL_PROC/3(MNSEG3)
  MNSEG4/1 -> OL_PROC/4(MNSEG4)
  Demux1/1 -> IPLo/1
  Demux1/2 -> IPTo/1
  Demux1/3 -> IPVo/1
  Demux1/4 -> IPRo/1
  Demux1/5 -> IPPo/1
  Demux1/6 -> IPYo/1
  Demux1/7 -> BFLo/1
  Demux1/8 -> BFTo/1
  Demux1/9 -> BFVo/1
  Demux1/10 -> BFRo/1
  Demux1/11 -> BFPo/1
  Demux1/12 -> BFYo/1
  Demux1/13 -> MNLo/1
  Demux1/14 -> MNTo/1
  Demux1/15 -> MNVo/1
  Demux1/16 -> MNRo/1
  Demux1/17 -> MNPo/1
  Demux1/18 -> MNYo/1
  Demux1/19 -> IMLo/1
  Demux1/20 -> IMTo/1
  Demux1/21 -> IMVo/1
  Demux1/22 -> IMRo/1
  Demux1/23 -> IMPo/1
  Demux1/24 -> IMYo/1
  Demux1/25 -> TMLo/1
  Demux1/26 -> TMTo/1
  Demux1/27 -> TMVo/1
  Demux1/28 -> TMRo/1
  Demux1/29 -> TMPop/1
  Demux1/30 -> TMYo/1
  F0/1 -> SENSIN_GAS/1(iF0)
  F1/1 -> SENSIN_GAS/2(iF1)
  F2/1 -> SENSIN_GAS/3(iF2)
  F3/1 -> SENSIN_GAS/4(iF3)
  BF/1 -> SENSIN_GAS/5(iBF)
  SEN2EUL_GAS/1 -> Demux6/1
  Mux6/1 -> SEN2EUL_GAS/1
  SENSIN_GAS/1(oF0) -> GAS_F0/1, Mux6/1
  SENSIN_GAS/2(oF1) -> GAS_F1/1, Mux6/2
  SENSIN_GAS/3(oF2) -> GAS_F2/1, Mux6/3
  SENSIN_GAS/4(oF3) -> GAS_F3/1, Mux6/4
  SENSIN_GAS/5(oBF) -> GAS_BF/1, Mux6/5
  DECPL_GAS/1 -> Demux3/1
  Mux1/1 -> DECPL_GAS/1
  Demux3/1 -> Mux3/1
  Demux3/2 -> Mux3/2
  Demux3/3 -> Mux3/3
  Demux3/4 -> Mux3/4
  Demux3/5 -> Mux3/5
  Mux3/1 -> Demux2/1
  SEN2EUL/1(IPLo) -> EUL/1(In1)
  SEN2EUL/2(IPTo) -> EUL/2(In2)
  SEN2EUL/3(IPVo) -> EUL/3(In3)
  SEN2EUL/4(IPRo) -> EUL/4(In4)
  SEN2EUL/5(IPPo) -> EUL/5(In5)
  SEN2EUL/6(IPYo) -> EUL/6(In6)
  SEN2EUL/7(BFLo) -> EUL/7(In7)
  SEN2EUL/8(BFTo) -> EUL/8(In8)
  SEN2EUL/9(BFVo) -> EUL/9(In9)
  SEN2EUL/10(BFRo) -> EUL/10(In10)
  SEN2EUL/11(BFPo) -> EUL/11(In11)
  SEN2EUL/12(BFYo) -> EUL/12(In12)
  SEN2EUL/13(MNLo) -> EUL/13(In13)
  SEN2EUL/14(MNTo) -> EUL/14(In14)
  SEN2EUL/15(MNVo) -> EUL/15(In15)
  SEN2EUL/16(MNRo) -> EUL/16(In16)
  SEN2EUL/17(MNPo) -> EUL/17(In17)
  SEN2EUL/18(MNYo) -> EUL/18(In18)
  SEN2EUL/19(IMLo) -> EUL/19(In19)
  SEN2EUL/20(IMTo) -> EUL/20(In20)
  SEN2EUL/21(IMVo) -> EUL/21(In21)
  SEN2EUL/22(IMRo) -> EUL/22(In22)
  SEN2EUL/23(IMPo) -> EUL/23(In23)
  SEN2EUL/24(IMYo) -> EUL/24(In24)
  SEN2EUL/25(TMLo) -> EUL/25(In25)
  SEN2EUL/26(TMTo) -> EUL/26(In26)
  SEN2EUL/27(TMVo) -> EUL/27(In27)
  SEN2EUL/28(TMRo) -> EUL/28(In28)
  SEN2EUL/29(TMPop) -> EUL/29(In29)
  SEN2EUL/30(TMYo) -> EUL/30(In30)
  EUL/1(Out1) -> DECPL/1(In1)
  EUL/2(Out2) -> DECPL/2(In2)
  EUL/3(Out3) -> DECPL/3(In3)
  EUL/4(Out4) -> DECPL/4(In4)
  EUL/5(Out5) -> DECPL/5(In5)
  EUL/6(Out6) -> DECPL/6(In6)
  EUL/7(Out7) -> DECPL/7(In7)
  EUL/8(Out8) -> DECPL/8(In8)
  EUL/9(Out9) -> DECPL/9(In9)
  EUL/10(Out10) -> DECPL/10(In10)
  EUL/11(Out11) -> DECPL/11(In11)
  EUL/12(Out12) -> DECPL/12(In12)
  EUL/13(Out13) -> DECPL/13(In13)
  EUL/14(Out14) -> DECPL/14(In14)
  EUL/15(Out15) -> DECPL/15(In15)
  EUL/16(Out16) -> DECPL/16(In16)
  EUL/17(Out17) -> DECPL/17(In17)
  EUL/18(Out18) -> DECPL/18(In18)
  EUL/19(Out19) -> DECPL/19(In27)
  EUL/20(Out20) -> DECPL/20(In28)
  EUL/21(Out21) -> DECPL/21(In29)
  EUL/22(Out22) -> DECPL/22(In30)
  EUL/23(Out23) -> DECPL/23(In31)
  EUL/24(Out24) -> DECPL/24(In32)
  EUL/25(Out25) -> DECPL/25(In33)
  EUL/26(Out26) -> DECPL/26(In34)
  EUL/27(Out27) -> DECPL/27(In35)
  EUL/28(Out28) -> DECPL/28(In36)
  EUL/29(Out29) -> DECPL/29(In37)
  EUL/30(Out30) -> DECPL/30(In38)
  Demux6/1 -> EUL_GAS/1
  Demux6/2 -> EUL_GAS/2
  Demux6/3 -> EUL_GAS/3
  Demux6/4 -> EUL_GAS/4
  Demux6/5 -> EUL_GAS/5
  EUL_GAS/1 -> Mux1/1
  EUL_GAS/2 -> Mux1/2
  EUL_GAS/3 -> Mux1/3
  EUL_GAS/4 -> Mux1/4
  EUL_GAS/5 -> Mux1/5
  SENSIN/1(IPV1) -> SEN2EUL/1(In1)
  SENSIN/2(IPV2) -> SEN2EUL/2(In2)
  SENSIN/3(IPV3) -> SEN2EUL/3(In3)
  SENSIN/4(IPH1) -> SEN2EUL/4(In4)
  SENSIN/5(IPH2) -> SEN2EUL/5(In5)
  SENSIN/6(IPH3) -> SEN2EUL/6(In6)
  SENSIN/7(BFV1) -> SEN2EUL/7(In7)
  SENSIN/8(BFV2) -> SEN2EUL/8(In8)
  SENSIN/9(BFV3) -> SEN2EUL/9(In9)
  SENSIN/10(BFH1) -> SEN2EUL/10(In10)
  SENSIN/11(BFH2) -> SEN2EUL/11(In11)
  SENSIN/12(BFH3) -> SEN2EUL/12(In12)
  SENSIN/13(MNV1) -> SEN2EUL/13(In13)
  SENSIN/14(MNV2) -> SEN2EUL/14(In14)
  SENSIN/15(MNV3) -> SEN2EUL/15(In15)
  SENSIN/16(MNH1) -> SEN2EUL/16(In20)
  SENSIN/17(MNH2) -> SEN2EUL/17(In21)
  SENSIN/18(MNH3) -> SEN2EUL/18(In22)
  SENSIN/19(IMV1) -> SEN2EUL/19(In27)
  SENSIN/20(IMV2) -> SEN2EUL/20(In28)
  SENSIN/21(IMV3) -> SEN2EUL/21(In29)
  SENSIN/22(IMH1) -> SEN2EUL/22(In30)
  SENSIN/23(IMH2) -> SEN2EUL/23(In31)
  SENSIN/24(IMH3) -> SEN2EUL/24(In32)
  SENSIN/25(IMV4) -> SEN2EUL/25(In33)
  SENSIN/26(IMV5) -> SEN2EUL/26(In34)
  SENSIN/27(IMV6) -> SEN2EUL/27(In35)
  SENSIN/28(IMH4) -> SEN2EUL/28(In36)
  SENSIN/29(IMH5) -> SEN2EUL/29(In37)
  SENSIN/30(IMH6) -> SEN2EUL/30(In38)
  SENSIN/31(MNOLV1) -> SEN2EUL/31(In16)
  SENSIN/32(MNOLV2) -> SEN2EUL/32(In17)
  SENSIN/33(MNOLV3) -> SEN2EUL/33(In18)
  SENSIN/34(MNOLH1) -> SEN2EUL/34(In19)
  SENSIN/35(MNOLH2) -> SEN2EUL/35(In23)
  SENSIN/36(MNOLH3) -> SEN2EUL/36(In24)
  SEN2EUL/31(TMLo1) -> EUL/31(In31)
  SEN2EUL/32(TMTo1) -> EUL/32(In32)
  SEN2EUL/33(TMVo1) -> EUL/33(In33)
  SEN2EUL/34(TMRo1) -> EUL/34(In34)
  SEN2EUL/35(TMPop1) -> EUL/35(In35)
  SEN2EUL/36(TMYo1) -> EUL/36(In36)
  EUL/31(Out31) -> DECPL/31(In19)
  EUL/32(Out32) -> DECPL/32(In20)
  EUL/33(Out33) -> DECPL/33(In21)
  EUL/34(Out34) -> DECPL/34(In22)
  EUL/35(Out35) -> DECPL/35(In23)
  EUL/36(Out36) -> DECPL/36(In24)
  Demux2/1 -> Mux2/37
  Demux2/2 -> Mux2/38
  Demux2/3 -> Mux2/39
  Demux2/4 -> Mux2/40
  Demux2/5 -> Mux2/41
  Demux1/37 -> GAS_M1/1
  Demux1/38 -> GAS_M2/1
  Demux1/39 -> GAS_M3/1
  Demux1/40 -> GAS_M4/1
  Demux1/41 -> GAS_M5/1
  Demux1/31 -> MNOLLo/1
  Demux1/32 -> MNOLTo/1
  Demux1/33 -> MNOLVo/1
  Demux1/34 -> MNOLRo/1
  Demux1/35 -> MNOLPo/1
  Demux1/36 -> MNOLYo/1
  DECPL/1(IPLo) -> Mux2/1
  DECPL/2(IPTo) -> Mux2/2
  DECPL/3(IPVo) -> Mux2/3
  DECPL/4(IPRo) -> Mux2/4
  DECPL/5(IPPo) -> Mux2/5
  DECPL/6(IPYo) -> Mux2/6
  DECPL/7(BFLo) -> Mux2/7
  DECPL/8(BFTo) -> Mux2/8
  DECPL/9(BFVo) -> Mux2/9
  DECPL/10(BFRo) -> Mux2/10
  DECPL/11(BFPo) -> Mux2/11
  DECPL/12(BFYo) -> Mux2/12
  DECPL/13(MNLo) -> Mux2/13
  DECPL/14(MNTo) -> Mux2/14
  DECPL/15(MNVo) -> Mux2/15
  DECPL/16(MNRo) -> Mux2/16
  DECPL/17(MNPo) -> Mux2/17
  DECPL/18(MNYo) -> Mux2/18
  DECPL/19(IMLo) -> Mux2/19
  DECPL/20(IMTo) -> Mux2/20
  DECPL/21(IMVo) -> Mux2/21
  DECPL/22(IMRo) -> Mux2/22
  DECPL/23(IMPo) -> Mux2/23
  DECPL/24(IMYo) -> Mux2/24
  DECPL/25(TMLo) -> Mux2/25
  DECPL/26(TMTo) -> Mux2/26
  DECPL/27(TMVo) -> Mux2/27
  DECPL/28(TMRo) -> Mux2/28
  DECPL/29(TMPop) -> Mux2/29
  DECPL/30(TMYo) -> Mux2/30
  DECPL/31(MNOLLo) -> Mux2/31
  DECPL/32(MNOLTo) -> Mux2/32
  DECPL/33(MNOLVo) -> Mux2/33
  DECPL/34(MNOLRo) -> Mux2/34
  DECPL/35(MNOLPo) -> Mux2/35
  DECPL/36(MNOLYo) -> Mux2/36
  Demux4/1 -> CAL/1(In1)
  Demux4/2 -> CAL/2(In2)
  Demux4/3 -> CAL/3(In3)
  Demux4/4 -> CAL/4(In4)
  Demux4/5 -> CAL/5(In5)
  Demux4/6 -> CAL/6(In6)
  Demux4/7 -> CAL/7(In7)
  Demux4/8 -> CAL/8(In8)
  Demux4/9 -> CAL/9(In9)
  Demux4/10 -> CAL/10(In10)
  Demux4/11 -> CAL/11(In11)
  Demux4/12 -> CAL/12(In12)
  Demux4/13 -> CAL/13(In13)
  Demux4/14 -> CAL/14(In14)
  Demux4/15 -> CAL/15(In15)
  Demux4/16 -> CAL/16(In16)
  Demux4/17 -> CAL/17(In17)
  Demux4/18 -> CAL/18(In18)
  Demux4/19 -> CAL/19(In19)
  Demux4/20 -> CAL/20(In20)
  Demux4/21 -> CAL/21(In21)
  Demux4/22 -> CAL/22(In22)
  Demux4/23 -> CAL/23(In23)
  Demux4/24 -> CAL/24(In24)
  Demux4/25 -> CAL/25(In25)
  Demux4/26 -> CAL/26(In26)
  Demux4/27 -> CAL/27(In27)
  Demux4/28 -> CAL/28(In28)
  Demux4/29 -> CAL/29(In29)
  Demux4/30 -> CAL/30(In30)
  Demux4/31 -> CAL/31(In31)
  Demux4/32 -> CAL/32(In32)
  Demux4/33 -> CAL/33(In33)
  Demux4/34 -> CAL/34(In34)
  Demux4/35 -> CAL/35(In35)
  Demux4/36 -> CAL/36(In36)
  Demux4/37 -> CAL/37(In37)
  Demux4/38 -> CAL/38(In38)
  Demux4/39 -> CAL/39(In39)
  Demux4/40 -> CAL/40(In40)
  Demux4/41 -> CAL/41(In41)
  Mux2/1 -> Demux1/1, Demux4/1
  CAL/1(Out1) -> Terminator/1
  CAL/2(Out2) -> Terminator1/1
  CAL/3(Out3) -> Terminator2/1
  CAL/4(Out4) -> Terminator3/1
  CAL/5(Out5) -> Terminator4/1
  CAL/6(Out6) -> Terminator5/1
  CAL/7(Out7) -> Terminator6/1
  CAL/8(Out8) -> Terminator7/1
  CAL/9(Out9) -> Terminator8/1
  CAL/10(Out10) -> Terminator9/1
  CAL/11(Out11) -> Terminator10/1
  CAL/12(Out12) -> Terminator11/1
  CAL/13(Out13) -> Terminator12/1
  CAL/14(Out14) -> Terminator13/1
  CAL/15(Out15) -> Terminator14/1
  CAL/16(Out16) -> Terminator15/1
  CAL/17(Out17) -> Terminator16/1
  CAL/18(Out18) -> Terminator17/1
  CAL/19(Out19) -> Terminator18/1
  CAL/20(Out20) -> Terminator19/1
  CAL/21(Out21) -> Terminator20/1
  CAL/22(Out22) -> Terminator21/1
  CAL/23(Out23) -> Terminator22/1
  CAL/24(Out24) -> Terminator23/1
  CAL/25(Out25) -> Terminator24/1
  CAL/26(Out26) -> Terminator25/1
  CAL/27(Out27) -> Terminator26/1
  CAL/28(Out28) -> Terminator27/1
  CAL/29(Out29) -> Terminator28/1
  CAL/30(Out30) -> Terminator29/1
  CAL/31(Out31) -> Terminator30/1
  CAL/32(Out32) -> Terminator31/1
  CAL/33(Out33) -> Terminator32/1
  CAL/34(Out34) -> Terminator33/1
  CAL/35(Out35) -> Terminator34/1
  CAL/36(Out36) -> Terminator35/1
  CAL/37(Out37) -> Terminator36/1
  CAL/38(Out38) -> Terminator37/1
  CAL/39(Out39) -> Terminator38/1
  CAL/40(Out40) -> Terminator39/1
  CAL/41(Out41) -> Terminator40/1

== system VIS_LIB/MODAL/sum ==
  In1 : Inport
  In2 : Inport  Port=2
  In3 : Inport  Port=3
  In4 : Inport  Port=4
  In5 : Inport  Port=5
  In6 : Inport  Port=6
  In7 : Inport  Port=7
  In8 : Inport  Port=8
  In9 : Inport  Port=9
  In10 : Inport  Port=10
  In11 : Inport  Port=11
  In12 : Inport  Port=12
  Sum : Sum  Inputs=++++++++++++
  Out1 : Outport
  wires:
  In2/1 -> Sum/2
  In10/1 -> Sum/10
  In8/1 -> Sum/8
  In12/1 -> Sum/12
  In1/1 -> Sum/1
  Sum/1 -> Out1/1
  In6/1 -> Sum/6
  In11/1 -> Sum/11
  In5/1 -> Sum/5
  In7/1 -> Sum/7
  In3/1 -> Sum/3
  In4/1 -> Sum/4
  In9/1 -> Sum/9

== system VIS_LIB/MODAL/sum1 ==
  In1 : Inport
  In12 : Inport  Port=2
  Sum : Sum
  Out1 : Outport
  wires:
  Sum/1 -> Out1/1
  In12/1 -> Sum/1
  In1/1 -> Sum/2

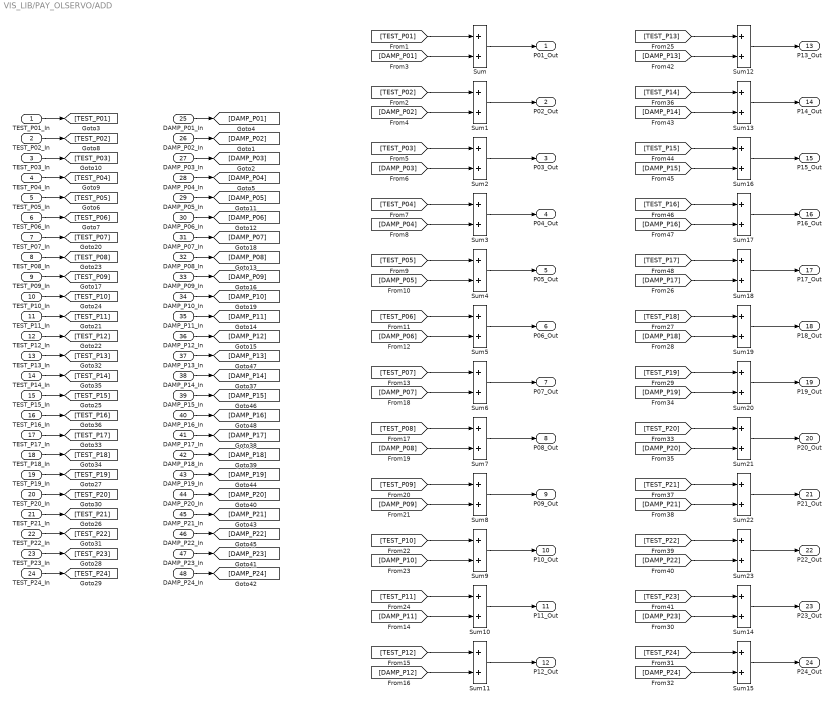
== system VIS_LIB/PAY_OLSERVO/ADD ==
  TEST_P01_In : Inport
  TEST_P02_In : Inport  Port=2
  TEST_P03_In : Inport  Port=3
  TEST_P04_In : Inport  Port=4
  TEST_P05_In : Inport  Port=5
  TEST_P06_In : Inport  Port=6
  TEST_P07_In : Inport  Port=7
  TEST_P08_In : Inport  Port=8
  TEST_P09_In : Inport  Port=9
  TEST_P10_In : Inport  Port=10
  TEST_P11_In : Inport  Port=11
  TEST_P12_In : Inport  Port=12
  TEST_P13_In : Inport  Port=13
  TEST_P14_In : Inport  Port=14
  TEST_P15_In : Inport  Port=15
  TEST_P16_In : Inport  Port=16
  TEST_P17_In : Inport  Port=17
  TEST_P18_In : Inport  Port=18
  TEST_P19_In : Inport  Port=19
  TEST_P20_In : Inport  Port=20
  TEST_P21_In : Inport  Port=21
  TEST_P22_In : Inport  Port=22
  TEST_P23_In : Inport  Port=23
  TEST_P24_In : Inport  Port=24
  DAMP_P01_In : Inport  Port=25
  DAMP_P02_In : Inport  Port=26
  DAMP_P03_In : Inport  Port=27
  DAMP_P04_In : Inport  Port=28
  DAMP_P05_In : Inport  Port=29
  DAMP_P06_In : Inport  Port=30
  DAMP_P07_In : Inport  Port=31
  DAMP_P08_In : Inport  Port=32
  DAMP_P09_In : Inport  Port=33
  DAMP_P10_In : Inport  Port=34
  DAMP_P11_In : Inport  Port=35
  DAMP_P12_In : Inport  Port=36
  DAMP_P13_In : Inport  Port=37
  DAMP_P14_In : Inport  Port=38
  DAMP_P15_In : Inport  Port=39
  DAMP_P16_In : Inport  Port=40
  DAMP_P17_In : Inport  Port=41
  DAMP_P18_In : Inport  Port=42
  DAMP_P19_In : Inport  Port=43
  DAMP_P20_In : Inport  Port=44
  DAMP_P21_In : Inport  Port=45
  DAMP_P22_In : Inport  Port=46
  DAMP_P23_In : Inport  Port=47
  DAMP_P24_In : Inport  Port=48
  Sum{,1..23} (24 alike) : Sum
  P01_Out : Outport
  P02_Out : Outport  Port=2
  P03_Out : Outport  Port=3
  P04_Out : Outport  Port=4
  P05_Out : Outport  Port=5
  P06_Out : Outport  Port=6
  P07_Out : Outport  Port=7
  P08_Out : Outport  Port=8
  P09_Out : Outport  Port=9
  P10_Out : Outport  Port=10
  P11_Out : Outport  Port=11
  P12_Out : Outport  Port=12
  P13_Out : Outport  Port=13
  P14_Out : Outport  Port=14
  P15_Out : Outport  Port=15
  P16_Out : Outport  Port=16
  P17_Out : Outport  Port=17
  P18_Out : Outport  Port=18
  P19_Out : Outport  Port=19
  P20_Out : Outport  Port=20
  P21_Out : Outport  Port=21
  P22_Out : Outport  Port=22
  P23_Out : Outport  Port=23
  P24_Out : Outport  Port=24
  wires:
  DAMP_P02_In/1 -> [DAMP_P02]
  DAMP_P01_In/1 -> [DAMP_P01]
  [DAMP_P01] -> Sum/2
  [TEST_P01] -> Sum/1
  Sum/1 -> P01_Out/1
  DAMP_P03_In/1 -> [DAMP_P03]
  TEST_P01_In/1 -> [TEST_P01]
  TEST_P02_In/1 -> [TEST_P02]
  TEST_P03_In/1 -> [TEST_P03]
  TEST_P04_In/1 -> [TEST_P04]
  TEST_P05_In/1 -> [TEST_P05]
  TEST_P06_In/1 -> [TEST_P06]
  DAMP_P05_In/1 -> [DAMP_P05]
  DAMP_P04_In/1 -> [DAMP_P04]
  DAMP_P06_In/1 -> [DAMP_P06]
  DAMP_P08_In/1 -> [DAMP_P08]
  DAMP_P07_In/1 -> [DAMP_P07]
  DAMP_P09_In/1 -> [DAMP_P09]
  DAMP_P11_In/1 -> [DAMP_P11]
  DAMP_P10_In/1 -> [DAMP_P10]
  DAMP_P12_In/1 -> [DAMP_P12]
  TEST_P07_In/1 -> [TEST_P07]
  TEST_P08_In/1 -> [TEST_P08]
  TEST_P09_In/1 -> [TEST_P09]
  TEST_P10_In/1 -> [TEST_P10]
  TEST_P11_In/1 -> [TEST_P11]
  TEST_P12_In/1 -> [TEST_P12]
  [DAMP_P02] -> Sum1/2
  [TEST_P02] -> Sum1/1
  Sum1/1 -> P02_Out/1
  [DAMP_P03] -> Sum2/2
  [TEST_P03] -> Sum2/1
  Sum2/1 -> P03_Out/1
  [DAMP_P04] -> Sum3/2
  [TEST_P04] -> Sum3/1
  Sum3/1 -> P04_Out/1
  [DAMP_P05] -> Sum4/2
  [TEST_P05] -> Sum4/1
  Sum4/1 -> P05_Out/1
  [DAMP_P06] -> Sum5/2
  [TEST_P06] -> Sum5/1
  Sum5/1 -> P06_Out/1
  [DAMP_P07] -> Sum6/2
  [TEST_P07] -> Sum6/1
  Sum6/1 -> P07_Out/1
  [DAMP_P08] -> Sum7/2
  [TEST_P08] -> Sum7/1
  Sum7/1 -> P08_Out/1
  [DAMP_P09] -> Sum8/2
  [TEST_P09] -> Sum8/1
  Sum8/1 -> P09_Out/1
  [DAMP_P10] -> Sum9/2
  [TEST_P10] -> Sum9/1
  Sum9/1 -> P10_Out/1
  [DAMP_P11] -> Sum10/2
  [TEST_P11] -> Sum10/1
  Sum10/1 -> P11_Out/1
  [DAMP_P12] -> Sum11/2
  [TEST_P12] -> Sum11/1
  Sum11/1 -> P12_Out/1
  TEST_P13_In/1 -> [TEST_P13]
  TEST_P14_In/1 -> [TEST_P14]
  TEST_P15_In/1 -> [TEST_P15]
  TEST_P16_In/1 -> [TEST_P16]
  TEST_P17_In/1 -> [TEST_P17]
  TEST_P18_In/1 -> [TEST_P18]
  TEST_P19_In/1 -> [TEST_P19]
  TEST_P20_In/1 -> [TEST_P20]
  TEST_P21_In/1 -> [TEST_P21]
  TEST_P22_In/1 -> [TEST_P22]
  TEST_P23_In/1 -> [TEST_P23]
  TEST_P24_In/1 -> [TEST_P24]
  DAMP_P14_In/1 -> [DAMP_P14]
  DAMP_P13_In/1 -> [DAMP_P13]
  DAMP_P15_In/1 -> [DAMP_P15]
  DAMP_P17_In/1 -> [DAMP_P17]
  DAMP_P16_In/1 -> [DAMP_P16]
  DAMP_P18_In/1 -> [DAMP_P18]
  DAMP_P20_In/1 -> [DAMP_P20]
  DAMP_P19_In/1 -> [DAMP_P19]
  DAMP_P21_In/1 -> [DAMP_P21]
  DAMP_P23_In/1 -> [DAMP_P23]
  DAMP_P22_In/1 -> [DAMP_P22]
  DAMP_P24_In/1 -> [DAMP_P24]
  [DAMP_P13] -> Sum12/2
  [TEST_P13] -> Sum12/1
  Sum12/1 -> P13_Out/1
  [DAMP_P14] -> Sum13/2
  [TEST_P14] -> Sum13/1
  Sum13/1 -> P14_Out/1
  [DAMP_P15] -> Sum16/2
  [TEST_P15] -> Sum16/1
  Sum16/1 -> P15_Out/1
  [DAMP_P16] -> Sum17/2
  [TEST_P16] -> Sum17/1
  Sum17/1 -> P16_Out/1
  [DAMP_P17] -> Sum18/2
  [TEST_P17] -> Sum18/1
  Sum18/1 -> P17_Out/1
  [DAMP_P18] -> Sum19/2
  [TEST_P18] -> Sum19/1
  Sum19/1 -> P18_Out/1
  [DAMP_P19] -> Sum20/2
  [TEST_P19] -> Sum20/1
  Sum20/1 -> P19_Out/1
  [DAMP_P20] -> Sum21/2
  [TEST_P20] -> Sum21/1
  Sum21/1 -> P20_Out/1
  [DAMP_P21] -> Sum22/2
  [TEST_P21] -> Sum22/1
  Sum22/1 -> P21_Out/1
  [DAMP_P22] -> Sum23/2
  [TEST_P22] -> Sum23/1
  Sum23/1 -> P22_Out/1
  [DAMP_P23] -> Sum14/2
  [TEST_P23] -> Sum14/1
  Sum14/1 -> P23_Out/1
  [DAMP_P24] -> Sum15/2
  [TEST_P24] -> Sum15/1
  Sum15/1 -> P24_Out/1
